simulink model "PBVS"  (Simulink 4.00)
settings: Solver=ode45  StartTime=0.0  StopTime=30.0  RelTol=1e-3
values from neighbouring files (symbols this model uses):
  c = camera(1000,1000,256,256,512,512)    [initHBVS.m]    (also in vsbrowser.m = handles.c)
  p = reshape(u,2,n)    [CamView.m]    (also in initHBVS.m = polyhedra([0.0 0.0 0; 0.25 0.25 0; -0.25 0.25 0; -0.25 -0.25; vsbrowser.m = handles.p)
  T0c_0 = T0c    [initHBVS.m]
  T0c_x = T0c    [initHBVS.m]
  T0o = handles.T0o    [vsbrowser.m]
undefined symbols (not defined in the file or in its folder): coords, get, GetHMatrix
libraries: vs x14
settings Model: LastModifiedBy=quique

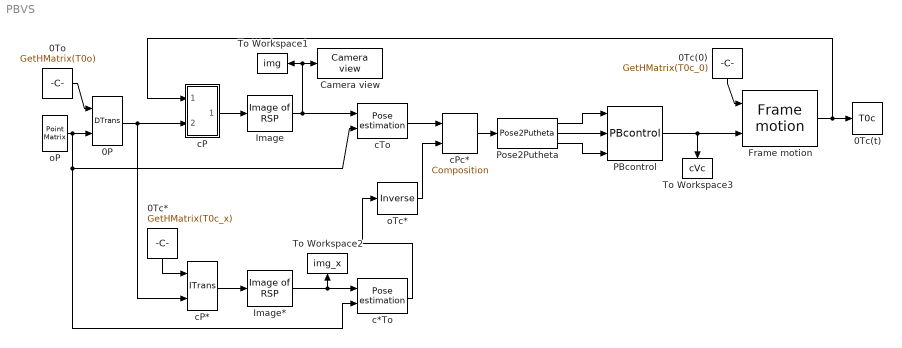
== system PBVS ==
  0P : vs/Features/DTrans
      settings: RTWFcnNameOpts=Auto  RTWFileNameOpts=Auto
  0Tc(0) : Constant  Orientation=down  Value=GetHMatrix(T0c_0)  VectorParams1D=off
  0Tc(t) : ToWorkspace  VariableName=T0c  SampleTime=-1  SaveFormat=StructureWithTime
  0Tc* : Constant  Orientation=down  Value=GetHMatrix(T0c_x)  VectorParams1D=off
  0To : Constant  Value=GetHMatrix(T0o)  VectorParams1D=off
  Camera view : vs/Camera/Camera view  ms=15  em=normal  umin=0  umax=get(c,'hres')-1  vmin=0  vmax=get(c,'vres')-1  st=-1
  Frame motion : vs/Pose/Frame motion
      settings: RTWFcnNameOpts=Auto  RTWFileNameOpts=Auto
  Image : vs/Camera/Image of RSP  fu=get(c,'fu')  fv=get(c,'fv')  u0=get(c,'u0')  v0=get(c,'v0')
  Image* : vs/Camera/Image of RSP  fu=get(c,'fu')  fv=get(c,'fv')  u0=get(c,'u0')  v0=get(c,'v0')
  PBcontrol : vs/Jacobian/PBcontrol  lambda=lambda
  Pose2Putheta : vs/Pose/Pose2Putheta
      settings: RTWFcnNameOpts=Auto  RTWFileNameOpts=Auto
  To Workspace1 : ToWorkspace  VariableName=img  SampleTime=-1  SaveFormat=StructureWithTime
  To Workspace2 : ToWorkspace  VariableName=img_x  SampleTime=-1  SaveFormat=StructureWithTime
      settings: Orientation=up
  To Workspace3 : ToWorkspace  VariableName=cVc  SampleTime=-1  SaveFormat=StructureWithTime
      settings: Orientation=down
  c*To : vs/Camera/Pose estimation  fu=get(c,'fu')  fv=get(c,'fv')  u0=get(c,'u0')  v0=get(c,'v0')  threshold=0.001
  cP : Subsystem  AncestorBlock=vs/Features/ITrans
      settings: RTWFcnNameOpts=Auto  RTWFileNameOpts=Auto
  cP* : vs/Features/ITrans
      settings: RTWFcnNameOpts=Auto  RTWFileNameOpts=Auto
  cPc* : vs/Pose/Composition
      settings: RTWFcnNameOpts=Auto  RTWFileNameOpts=Auto
  cTo : vs/Camera/Pose estimation  fu=get(c,'fu')  fv=get(c,'fv')  u0=get(c,'u0')  v0=get(c,'v0')  threshold=0.001
  oP : vs/Features/Point Matrix  m=coords(p)
  oTc* : vs/Pose/Inverse
      settings: RTWFcnNameOpts=Auto  RTWFileNameOpts=Auto
  wires:
  oP/1 -> 0P/2, c*To/2, cTo/2
  cP/1(bP) -> Image/1
  Image/1 -> Camera view/1, To Workspace1/1, cTo/1
  Frame motion/1 -> 0Tc(t)/1, cP/1(aTb)
  0Tc*/1 -> cP*/1
  cP*/1 -> Image*/1
  0Tc(0)/1 -> Frame motion/1
  0To/1 -> 0P/1
  0P/1 -> cP/2(aP), cP*/2
  PBcontrol/1 -> Frame motion/2, To Workspace3/1
  Image*/1 -> To Workspace2/1, c*To/1
  c*To/1 -> oTc*/1
  cTo/1 -> cPc*/1
  oTc*/1 -> cPc*/2
  cPc*/1 -> Pose2Putheta/1
  Pose2Putheta/2 -> PBcontrol/2
  Pose2Putheta/1 -> PBcontrol/1
  Pose2Putheta/3 -> PBcontrol/3

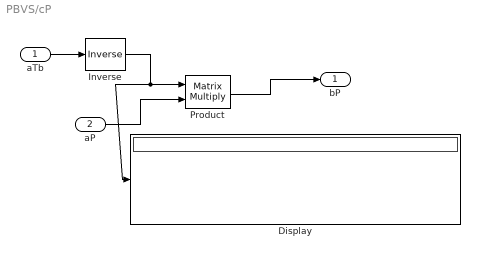
== system PBVS/cP ==
  aTb : Inport  Port=1  LatchInput=off
  aP : Inport  Port=2  LatchInput=off
  Display : Display
      settings: Format=short
  Inverse : vs/Pose/Inverse
      settings: RTWFcnNameOpts=Auto  RTWFileNameOpts=Auto
  Product : Product  Inputs=2  Multiplication=Matrix(*)  SaturateOnIntegerOverflow=on
  bP : Outport  Port=1
  wires:
  Inverse/1 -> Product/1, Display/1
  aTb/1 -> Inverse/1
  Product/1 -> bP/1
  aP/1 -> Product/2
